simulink model "lqr_control_kalman_observer_continuous"  (R2020b)
settings: Solver=VariableStepAuto  StartTime=0.0  StopTime=10.0  RelTol=1e-3
undefined symbols (not defined in the file): A, B, C, D, G, h, h_plant, L, measure_noise_covariance, process_noise_covariance, reference, sat_max, sat_min, wind_final_value, wind_initial_value, wind_steptime, x0, x0_observer
settings Model: Creator=lucas  LastModifiedBy=lucas

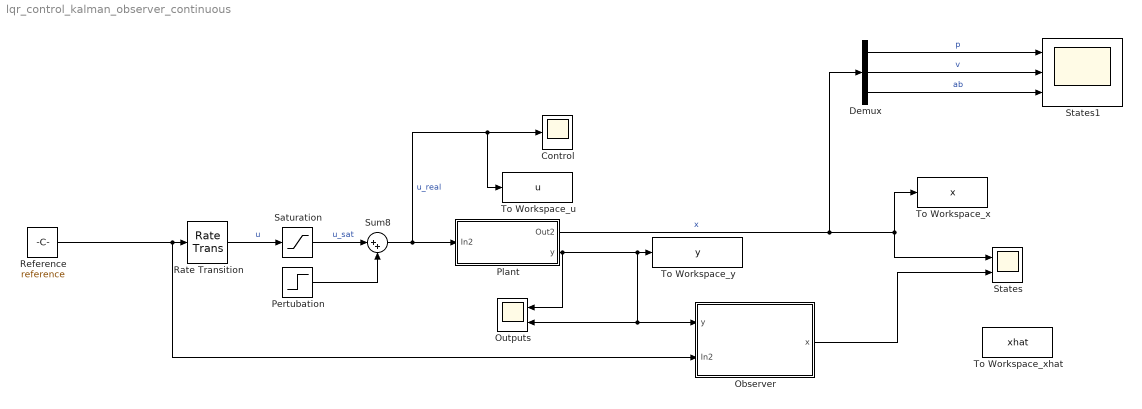
== system lqr_control_kalman_observer_continuous ==
  Control : Scope
  Demux : Demux  Outputs=3
  Observer : Subsystem
  Outputs : Scope  NumInputPorts=2
  Pertubation : Step  Time=wind_steptime  Before=wind_initial_value  After=wind_final_value  SampleTime=h_plant
  Plant : Subsystem
  Rate Transition : RateTransition  Integrity=off  OutPortSampleTimeMultiple=0.01  OutPortSampleTime=h_plant
  Reference : Constant  Value=reference  SampleTime=h
  Saturation : Saturate  UpperLimit=sat_max  LowerLimit=sat_min
  States : Scope  NumInputPorts=2
  States1 : Scope  NumInputPorts=3
  Sum8 : Sum  Inputs=|++
  To Workspace_u : ToWorkspace  VariableName=u  SaveFormat=Timeseries  SampleTime=-1
  To Workspace_x : ToWorkspace  VariableName=x  SaveFormat=Timeseries  SampleTime=-1
  To Workspace_xhat : ToWorkspace  VariableName=xhat  SaveFormat=Timeseries  SampleTime=-1
  To Workspace_y : ToWorkspace  VariableName=y  SaveFormat=Timeseries  SampleTime=-1
  wires:
  Rate Transition/1 -> Saturation/1  "u"
  Plant/2(y) -> Outputs/1, Observer/1(y), Outputs/2, To Workspace_y/1
  Pertubation/1 -> Sum8/2
  Saturation/1 -> Sum8/1  "u_sat"
  Plant/1(Out2) -> Demux/1, To Workspace_x/1, States/1  "x"
  Reference/1 -> Observer/2(In2), Rate Transition/1
  Sum8/1 -> Plant/1(In2), To Workspace_u/1, Control/1  "u_real"
  Observer/1(x) -> States/2
  Demux/1 -> States1/1  "p"
  Demux/2 -> States1/2  "v"
  Demux/3 -> States1/3  "ab"

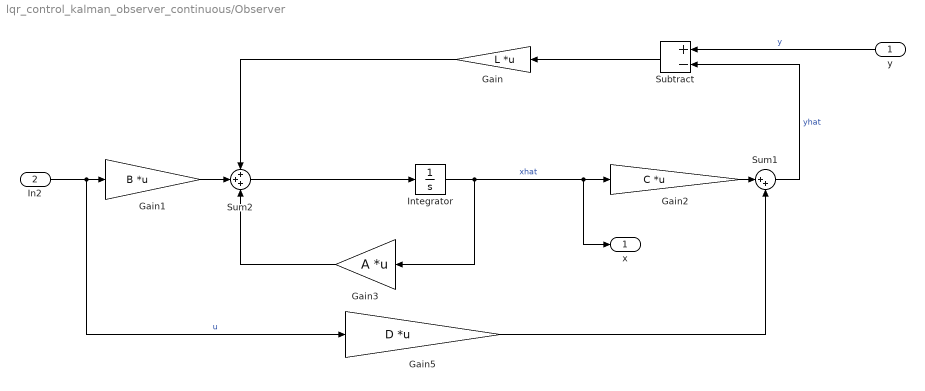
== system lqr_control_kalman_observer_continuous/Observer ==
  y : Inport
  In2 : Inport  Port=2
  Gain : Gain  Gain=L  Multiplication=Matrix(K*u) (u vector)
  Gain1 : Gain  Gain=B  Multiplication=Matrix(K*u) (u vector)
  Gain2 : Gain  Gain=C  Multiplication=Matrix(K*u) (u vector)
  Gain3 : Gain  Gain=A  Multiplication=Matrix(K*u) (u vector)
  Gain5 : Gain  Gain=D  Multiplication=Matrix(K*u) (u vector)
  Integrator : Integrator  InitialCondition=x0_observer
  Subtract : Sum  Inputs=+-
  Sum1 : Sum  Inputs=|++
  Sum2 : Sum  Inputs=+++
  x : Outport
  wires:
  Gain5/1 -> Sum1/2
  In2/1 -> Gain5/1, Gain1/1  "u"
  Sum2/1 -> Integrator/1
  Gain3/1 -> Sum2/3
  Integrator/1 -> Gain3/1, x/1, Gain2/1  "xhat"
  Gain1/1 -> Sum2/2
  Gain2/1 -> Sum1/1
  y/1 -> Subtract/1  "y"
  Sum1/1 -> Subtract/2  "yhat"
  Subtract/1 -> Gain/1
  Gain/1 -> Sum2/1

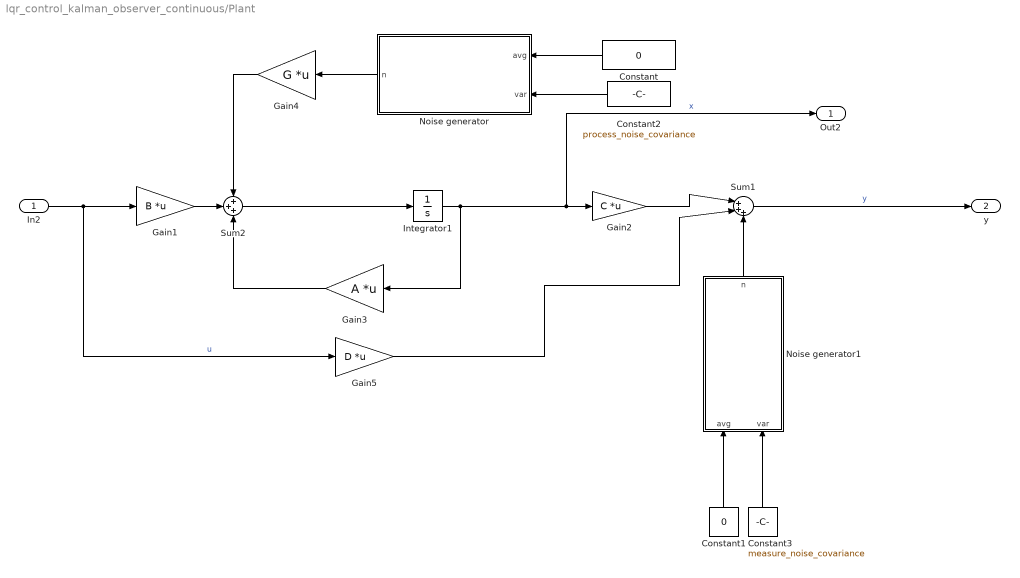
== system lqr_control_kalman_observer_continuous/Plant ==
  In2 : Inport
  Constant : Constant  Value=0  VectorParams1D=off
  Constant1 : Constant  Value=0
  Constant2 : Constant  Value=process_noise_covariance
  Constant3 : Constant  Value=measure_noise_covariance
  Gain1 : Gain  Gain=B  Multiplication=Matrix(K*u) (u vector)
  Gain2 : Gain  Gain=C  Multiplication=Matrix(K*u) (u vector)
  Gain3 : Gain  Gain=A  Multiplication=Matrix(K*u) (u vector)
  Gain4 : Gain  Gain=G  Multiplication=Matrix(K*u) (u vector)
  Gain5 : Gain  Gain=D  Multiplication=Matrix(K*u) (u vector)
  Integrator1 : Integrator  InitialCondition=x0
  Noise generator : MATLAB Function  TreatAsAtomicUnit=on
  Noise generator1 : MATLAB Function  TreatAsAtomicUnit=on
  Sum1 : Sum  Inputs=|+++
  Sum2 : Sum  Inputs=+++
  Out2 : Outport
  y : Outport  Port=2
  wires:
  Sum2/1 -> Integrator1/1
  Gain2/1 -> Sum1/1
  Sum1/1 -> y/1  "y"
  In2/1 -> Gain5/1, Gain1/1  "u"
  Integrator1/1 -> Gain3/1, Out2/1, Gain2/1  "x"
  Gain1/1 -> Sum2/2
  Gain3/1 -> Sum2/3
  Noise generator/1(n) -> Gain4/1
  Gain4/1 -> Sum2/1
  Constant/1 -> Noise generator/1(avg)
  Constant1/1 -> Noise generator1/1(avg)
  Constant3/1 -> Noise generator1/2(var)
  Constant2/1 -> Noise generator/2(var)
  Noise generator1/1(n) -> Sum1/3
  Gain5/1 -> Sum1/2

== matlab function lqr_control_kalman_observer_continuous/Plant/Noise generator ==
  data: avg input; n output; var input
function n = generate_gaussian_noise(avg, var)
n = avg + var*randn(length(var), 1);

== matlab function lqr_control_kalman_observer_continuous/Plant/Noise generator1 ==
  data: avg input; n output; var input
function n = generate_gaussian_noise(avg, var)
n = avg + var*randn(length(var), 1);
